simulink model "assumed_mode_wout_ps2f_simulink"  (R2025b)
settings: Solver=ode4  StartTime=0.0  StopTime=inf  FixedStep=0.02  RelTol=1e-3  EnableMultiTasking=on
values from neighbouring files (symbols this model uses):
  par = [ ... (first row only)    [build_ppo_parameter_vector.m]    (also in run_assumed_mode.m; test_ppo_ps2f_simulink.m = build_ppo_parameter_vector(p,Ts,2); test_ppo_simulink.m = build_ppo_parameter_vector(p,Ts,2); train_ppo_simulink.m = build_ppo_parameter_vector(p,Ts,2))
settings Model: ExtModeTrigDuration=10000  Creator=Nargiz  LastModifiedBy=Nargiz
settings SolverCC: AlgebraicLoopSolver=TrustRegion  PositivePriorityOrder=on
settings DataIOCC: ReturnWorkspaceOutputs=off
settings OptimizationCC: LifeSpan=inf
settings DebuggingCC: UnconnectedInputMsg=warning  UnconnectedOutputMsg=warning  UnconnectedLineMsg=warning  ArithmeticOperatorsInVariantConditions=warning
settings ModelReferenceCC: EnableRefExpFcnMdlSchedulingChecks=on
settings SFSimCC: SimUseLocalCustomCode=off  CustomCodeUndefinedFunction=UseInterfaceOnly
settings RTWCC: SystemTargetFile=quarc_win64.tlc  TemplateMakefile=quarc_default_tmf  RTWUseLocalCustomCode=off  GPUComputeCapability=3.5  Description=QUARC Win64 Target
settings CodeAppCC: StateflowObjectComments=on
settings STFCustomTargetCC: SystemTargetFile=quarc_win64.tlc  TargetPreCompLibLocation=C:\PROGRA~3\QUARC\lib\2016a\win64\release  TargetLangStandard=C99 (ISO)  StopOnOverrun=off  DownloadToTarget=on  Debug=off
settings GRTTargetCC: ExtMode=on  ExtModeMexFile=quarc_comm  TargetPreCompLibLocation=C:\PROGRA~3\QUARC\lib\2016a\win64\release  ParMdlRefBuildCompliant=off  CompOptLevelCompliant=off  CombineOutputUpdateFcns=off  MatFileLogging=off  CPPClassGenCompliant=off  GRTInterface=on  UseToolchainInfoCompliant=off
settings ConfigComp: CovMetricSettings=dswe

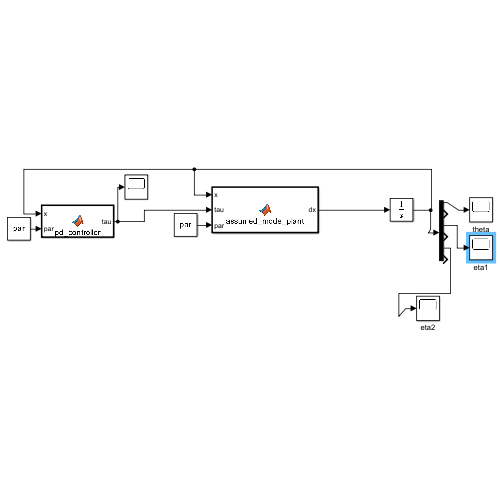
[thumbnail: Simulink's stored preview of the top-level diagram]
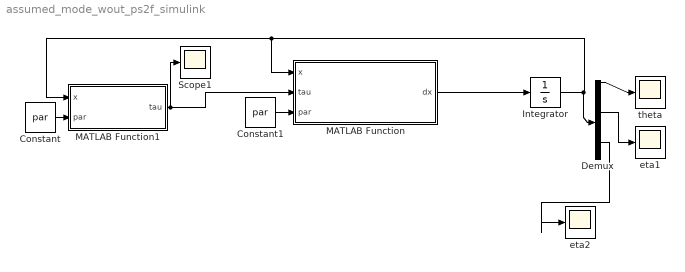
== system assumed_mode_wout_ps2f_simulink ==
  Constant : Constant  Value=par
  Constant1 : Constant  Value=par
  Demux : Demux  Outputs=6
  Integrator : Integrator
  MATLAB Function : MATLAB Function  TreatAsAtomicUnit=on
  MATLAB Function1 : MATLAB Function  TreatAsAtomicUnit=on
  Scope1 : Scope
      settings: ActiveDisplayYMinimum=-1  ActiveDisplayYMaximum=1
  eta1 : Scope
      settings: ActiveDisplayYMinimum=-0.0090806922733996237  ActiveDisplayYMaximum=0.010055002550571387  DataLoggingVariableName=ScopeData2
  eta2 : Scope
      settings: ActiveDisplayYMinimum=-0.00026217163202578583  ActiveDisplayYMaximum=0.00052299781344427492  DataLoggingVariableName=ScopeData3
  theta : Scope
      settings: ActiveDisplayYMinimum=-0.065798320813010652  ActiveDisplayYMaximum=0.592184887317096
  wires:
  Integrator/1 -> Demux/1, MATLAB Function/1(x), MATLAB Function1/1(x)
  MATLAB Function/1(dx) -> Integrator/1
  Demux/3 -> eta1/1
  Demux/1 -> theta/1
  Constant1/1 -> MATLAB Function/3(par)
  Demux/5 -> eta2/1
  Constant/1 -> MATLAB Function1/2(par)
  MATLAB Function1/1(tau) -> Scope1/1, MATLAB Function/2(tau)

== matlab function assumed_mode_wout_ps2f_simulink/MATLAB Function1 ==
  data: x input; tau output; par input
function tau = pd_controller(x, par)

theta     = x(1);
theta_dot = x(2);

Kp          = par(17);
Kd          = par(18);
theta_d     = par(19);
theta_dot_d = par(20);
tau_max     = par(21);

tau = -Kp*(theta - theta_d) - Kd*(theta_dot - theta_dot_d);

tau = max(min(tau, tau_max), -tau_max);

end

== matlab function assumed_mode_wout_ps2f_simulink/MATLAB Function ==
  data: x input; tau input; dx output; par input
function dx = assumed_mode_plant(x, tau, par)

%#codegen

dx = zeros(6,1);   % IMPORTANT: define output size immediately

%% Unpack parameter vector
l       = par(2);
J2      = par(3);
mr      = par(4);
mp      = par(5);
Btheta  = par(6);

phi1L   = par(7);
phi2L   = par(8);
phi1pL  = par(9);
phi2pL  = par(10);

Meta1   = par(11);
Meta2   = par(12);
Keta1   = par(13);
Keta2   = par(14);
Deta1   = par(15);
Deta2   = par(16);

tau_max = par(21);

%% States
theta     = x(1);
theta_dot = x(2);

eta1      = x(3);
eta1_dot  = x(4);

eta2      = x(5);
eta2_dot  = x(6);

qdot = [theta_dot; eta1_dot; eta2_dot];

%% Torque saturation
tau = max(min(tau, tau_max), -tau_max);

%% Tip deflection and tip slope
alpha = phi1pL*eta1 + phi2pL*eta2;
gamma = theta + alpha;

gvec = [1; phi1pL; phi2pL];
wvec = [0; phi1L; phi2L];

%% Rigid link and payload coefficients
Ir = mr*l^2/3;
Ip = mp*l^2;

Arot = Ir + Ip;
Mvert = mr + mp;
Across = mr*l/2 + mp*l;

%% Mass matrix
M = zeros(3,3);

M(1,1) = M(1,1) + J2;
M(2,2) = M(2,2) + Meta1;
M(3,3) = M(3,3) + Meta2;

M = M ...
    + Arot*(gvec*gvec') ...
    + Mvert*(wvec*wvec') ...
    + Across*cos(gamma)*(gvec*wvec' + wvec*gvec');

%% Nonlinear velocity terms
dM = zeros(3,3,3);

common_dM_dgamma = -Across*sin(gamma)*(gvec*wvec' + wvec*gvec');

for kk = 1:3
    dM(:,:,kk) = common_dM_dgamma * gvec(kk);
end

h = zeros(3,1);

for ii = 1:3
    for jj = 1:3
        for kk = 1:3
            Gamma_ijk = 0.5*(dM(ii,jj,kk) + dM(ii,kk,jj) - dM(jj,kk,ii));
            h(ii) = h(ii) + Gamma_ijk*qdot(jj)*qdot(kk);
        end
    end
end

%% Stiffness and damping
Kq = [0;
      Keta1*eta1;
      Keta2*eta2];

Dq = [Btheta*theta_dot;
      Deta1*eta1_dot;
      Deta2*eta2_dot];

Q = [tau; 0; 0];

%% Solve dynamics
qdd = M \ (Q - h - Dq - Kq);

%% Output derivative
dx(1) = theta_dot;
dx(2) = qdd(1);

dx(3) = eta1_dot;
dx(4) = qdd(2);

dx(5) = eta2_dot;
dx(6) = qdd(3);

end
